simulink model "goertzel_algorithm2"  (R2021b)
settings: Solver=FixedStepAuto  StartTime=0.0  StopTime=100.0  FixedStep=0.001  RelTol=1e-3
values from neighbouring files (symbols this model uses):
  coeff = 2*cos(omega)    [create_simulink_model.m]
  N = 1000    [create_simulink_model.m]
  omega = 2*pi*k/N    (= 0.0628318530718)    [create_simulink_model.m]
libraries: hdlsllib x2, simulink x1, commrandsrc3 x1
settings Model: Creator=caccolillo  LastModifiedBy=caccolillo

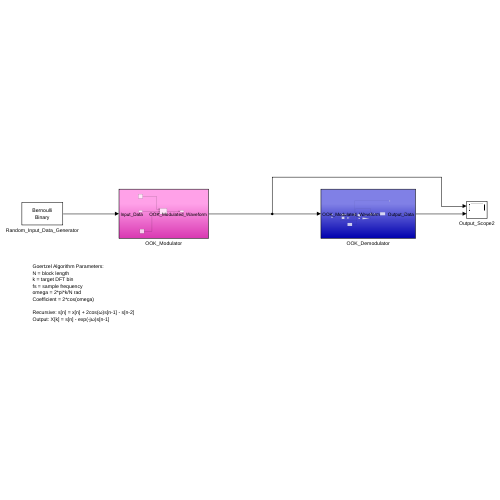
[thumbnail: Simulink's stored preview of the top-level diagram]
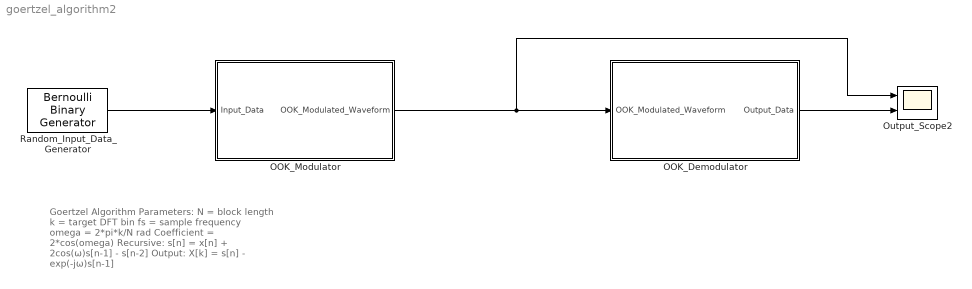
== system goertzel_algorithm2 ==
  note: Goertzel Algorithm Parameters:
      | N = block length
      | k = target DFT bin
      | fs = sample frequency
      | omega = 2*pi*k/N rad
      | Coefficient = 2*cos(omega)
      |
      | Recursive: s[n] = x[n] + 2cos(ω)s[n-1] - s[n-2]
      | Output: X[k] = s[n] - exp(-jω)s[n-1]
  OOK_Demodulator : Subsystem
  OOK_Modulator : Subsystem
  Output_Scope2 : Scope  NumInputPorts=2
  Random_Input_Data_Generator : commrandsrc3/Bernoulli Binary Generator  ProbabilityOfZero=0.5  SeedSource=Auto  Seed=0  SampleTime=1  SamplesPerFrame=1  OutputDataType=double  SimulateUsing=Interpreted execution
  wires:
  OOK_Modulator/1(OOK_Modulated_Waveform) -> OOK_Demodulator/1(OOK_Modulated_Waveform), Output_Scope2/1
  Random_Input_Data_Generator/1 -> OOK_Modulator/1(Input_Data)
  OOK_Demodulator/1(Output_Data) -> Output_Scope2/2

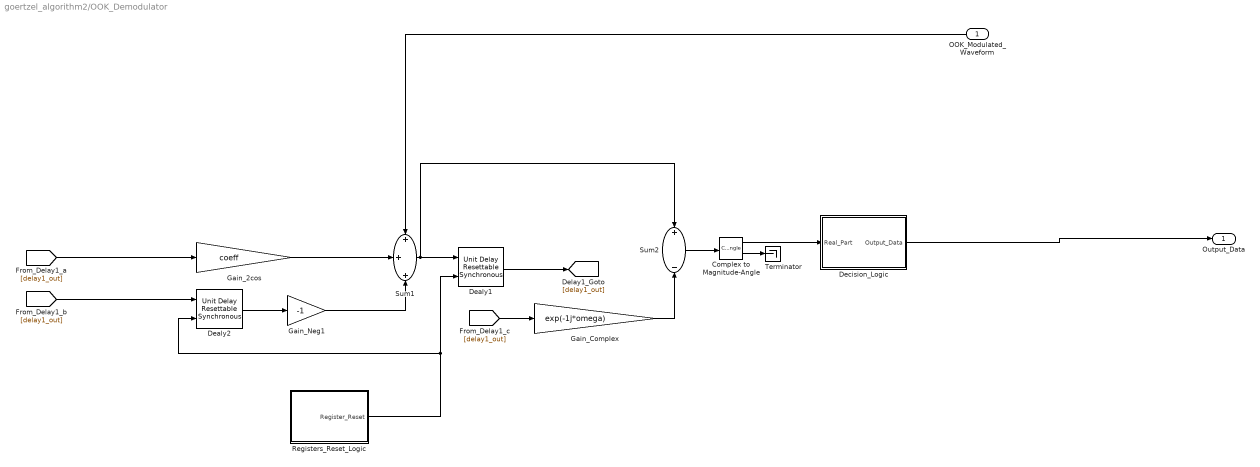
== system goertzel_algorithm2/OOK_Demodulator ==
  OOK_Modulated_Waveform : Inport
  Complex to Magnitude-Angle : ComplexToMagnitudeAngle
  Dealy1 : hdlsllib/Discrete/Unit Delay Resettable Synchronous  InitialCondition=0.0  SampleTime=-1
      settings: SourceProductBaseCode=SL
  Dealy2 : hdlsllib/Discrete/Unit Delay Resettable Synchronous  InitialCondition=0.0  SampleTime=-1
      settings: SourceProductBaseCode=SL
  Decision_Logic : Subsystem
  Gain_2cos : Gain  Gain=coeff
  Gain_Complex : Gain  Gain=exp(-1j*omega)
  Gain_Neg1 : Gain  Gain=-1
  Registers_Reset_Logic : Subsystem
  Sum1 : Sum  Inputs=+++
  Sum2 : Sum  Inputs=+-
  Terminator : Terminator
  Output_Data : Outport
  wires:
  Gain_Neg1/1 -> Sum1/3
  Gain_Complex/1 -> Sum2/2
  [delay1_out] -> Gain_Complex/1
  Dealy2/1 -> Gain_Neg1/1
  Dealy1/1 -> [delay1_out]
  Complex to Magnitude-Angle/2 -> Terminator/1
  [delay1_out] -> Gain_2cos/1
  Registers_Reset_Logic/1(Register_Reset) -> Dealy2/2, Dealy1/2
  OOK_Modulated_Waveform/1 -> Sum1/1
  Sum2/1 -> Complex to Magnitude-Angle/1
  [delay1_out] -> Dealy2/1
  Decision_Logic/1(Output_Data) -> Output_Data/1
  Sum1/1 -> Sum2/1, Dealy1/1
  Complex to Magnitude-Angle/1 -> Decision_Logic/1(Real_Part)
  Gain_2cos/1 -> Sum1/2

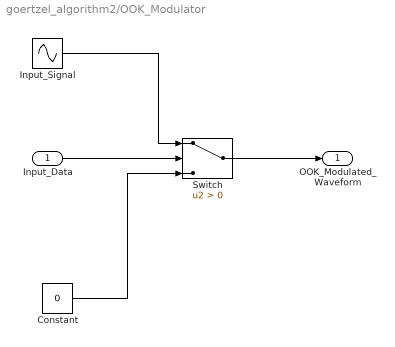
== system goertzel_algorithm2/OOK_Modulator ==
  Input_Data : Inport
  Constant : Constant  Value=0
  Input_Signal : Sin  Frequency=2*pi*50  SampleTime=0.001
  Switch : Switch  Criteria=u2 > Threshold
  OOK_Modulated_Waveform : Outport
  wires:
  Input_Data/1 -> Switch/2
  Input_Signal/1 -> Switch/1
  Switch/1 -> OOK_Modulated_Waveform/1
  Constant/1 -> Switch/3

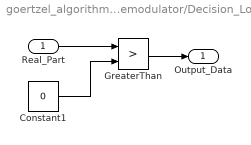
== system goertzel_algorithm2/OOK_Demodulator/Decision_Logic ==
  Real_Part : Inport
  Constant1 : Constant  Value=0
  GreaterThan : RelationalOperator  Operator=>  OutDataTypeStr=boolean  RndMeth=Simplest
  Output_Data : Outport
  wires:
  Constant1/1 -> GreaterThan/2
  Real_Part/1 -> GreaterThan/1
  GreaterThan/1 -> Output_Data/1

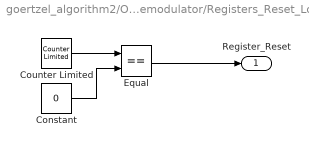
== system goertzel_algorithm2/OOK_Demodulator/Registers_Reset_Logic ==
  Constant : Constant  Value=0
  Counter Limited : simulink/Sources/Counter Limited  uplimit=N  tsamp=0.001
  Equal : RelationalOperator  Operator===  OutDataTypeStr=boolean  RndMeth=Simplest
  Register_Reset : Outport
  wires:
  Constant/1 -> Equal/2
  Counter Limited/1 -> Equal/1
  Equal/1 -> Register_Reset/1
